simulink model "s_jsj4_11"  (Simulink 5.0)
settings: Solver=ode45  SolverMode=SingleTasking  StartTime=0.0  StopTime=1  FixedStep=0.1  RelTol=1e-3
libraries: cstblocks x2, simulink_extras x1
settings Model: LastModifiedBy=ThinkPad

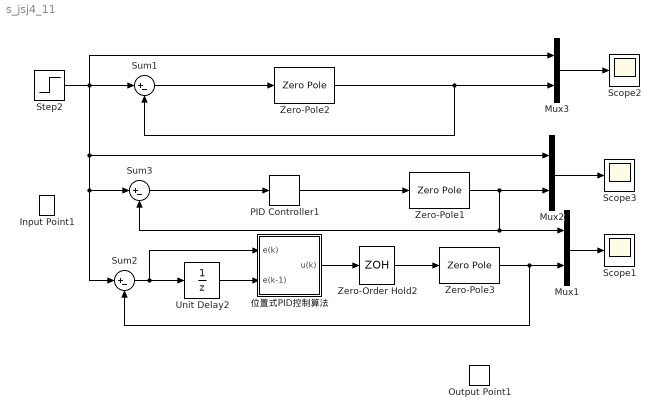
== system s_jsj4_11 ==
  Input Point1 : cstblocks/Input Point
  Mux1 : Mux  Inputs=2
  Mux2 : Mux  Inputs=2
  Mux3 : Mux  Inputs=2
  Output Point1 : cstblocks/Output Point
  PID Controller1 : simulink_extras/Additional Linear/PID Controller  P=8  I=0.05  D=0.4
  Scope1 : Scope
      settings: YMin=-3.5  YMax=1  MaxDataPoints=500000
  Scope2 : Scope
      settings: YMin=-3.5  YMax=1  MaxDataPoints=500000
  Scope3 : Scope
      settings: TimeRange=0.4000000000000001  YMin=1.01244  YMax=1.01585  SaveName=ScopeData2  MaxDataPoints=500000
  Step2 : Step  Time=0  SampleTime=0
  Sum1 : Sum  Inputs=|+-  SaturateOnIntegerOverflow=on
  Sum2 : Sum  Inputs=|+-  SaturateOnIntegerOverflow=on
  Sum3 : Sum  Inputs=|+-  SaturateOnIntegerOverflow=on
  Unit Delay2 : UnitDelay  SampleTime=0.001
  Zero-Order Hold2 : ZeroOrderHold  SampleTime=0.001
  Zero-Pole1 : ZeroPole  Zeros=[]  Poles=[0 -4]  Gain=[120]
  Zero-Pole2 : ZeroPole  Zeros=[]  Poles=[0 -4]  Gain=[120]
  Zero-Pole3 : ZeroPole  Zeros=[]  Poles=[0 -4]  Gain=[120]
  位置式PID控制算法 : Subsystem
  wires:
  Step2/1 -> Mux3/1, Sum1/1, Mux2/1, Sum3/1, Sum2/1
  Zero-Pole1/1 -> Mux2/2, Sum3/2, Mux1/1
  PID Controller1/1 -> Zero-Pole1/1
  Mux3/1 -> Scope2/1
  Sum1/1 -> Zero-Pole2/1
  Sum3/1 -> PID Controller1/1
  Zero-Pole2/1 -> Mux3/2, Sum1/2
  Mux2/1 -> Scope3/1
  位置式PID控制算法/1(u(k)) -> Zero-Order Hold2/1
  Sum2/1 -> 位置式PID控制算法/1(e(k)), Unit Delay2/1
  Unit Delay2/1 -> 位置式PID控制算法/2(e(k-1))
  Zero-Order Hold2/1 -> Zero-Pole3/1
  Zero-Pole3/1 -> Mux1/2, Sum2/2
  Mux1/1 -> Scope1/1

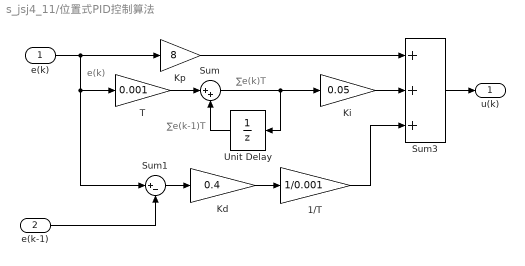
== system s_jsj4_11/位置式PID控制算法 ==
  note: e(k)
  note: ∑e(k)T
  note: ∑e(k-1)T
  e(k) : Inport
  e(k-1) : Inport  Port=2
  1/T : Gain  Gain=1/0.001  SaturateOnIntegerOverflow=on
  Kd : Gain  Gain=0.4  SaturateOnIntegerOverflow=on
  Ki : Gain  Gain=0.05  SaturateOnIntegerOverflow=on
  Kp : Gain  Gain=8  SaturateOnIntegerOverflow=on
  Sum : Sum  Inputs=|++  SaturateOnIntegerOverflow=on
  Sum1 : Sum  Inputs=|+-  SaturateOnIntegerOverflow=on
  Sum3 : Sum  Inputs=+++  SaturateOnIntegerOverflow=on
  T : Gain  Gain=0.001  SaturateOnIntegerOverflow=on
  Unit Delay : UnitDelay  Orientation=left  SampleTime=0.001
  u(k) : Outport
  wires:
  Sum1/1 -> Kd/1
  e(k)/1 -> Kp/1, Sum1/1, T/1
  Kp/1 -> Sum3/1
  Ki/1 -> Sum3/2
  Sum3/1 -> u(k)/1
  Kd/1 -> 1/T/1
  1/T/1 -> Sum3/3
  Sum/1 -> Unit Delay/1, Ki/1
  Unit Delay/1 -> Sum/2
  e(k-1)/1 -> Sum1/2
  T/1 -> Sum/1
